simulink model "artigo_pista"  (R2018a)
settings: Solver=ode45  StartTime=0.0  StopTime=6  RelTol=1e-5  EnableMultiTasking=on
undefined symbols (not defined in the file): KIm, Km, KPm, mapa_pista_artigo, Pm, Ts
libraries: simulink x4
settings Model: Creator=dwbertol  LastModifiedBy=bruno
settings DataIOCC: LimitDataPoints=on  SaveFormat=Array  SignalLoggingSaveFormat=ModelDataLogs
settings OptimizationCC: ExpressionDepthLimit=2147483647  LifeSpan=inf
settings DebuggingCC: UnderspecifiedInitializationDetection=Classic  MergeDetectMultiDrivingBlocksExec=none  SolverPrmCheckMsg=warning  FcnCallInpInsideContextMsg=warning  StateNameClashWarn=warning  SFUnexpectedBacktrackingDiag=warning  SFNoUnconditionalDefaultTransitionDiag=warning  SFExecutionAtInitializationDiag=none
settings HardwareCC: ProdBitPerPointer=32  ProdBitPerSizeT=32  ProdBitPerPtrDiffT=32  ProdLargestAtomicFloat=None  ProdIntDivRoundTo=Undefined  ProdEndianess=Unspecified  ProdWordSize=32  ProdHWDeviceType=32-bit Generic
settings ModelReferenceCC: PropagateSignalLabelsOutOfModel=off
settings CodeAppCC: StateflowObjectComments=on
settings GRTTargetCC: TargetLangStandard=C89/C90 (ANSI)  GeneratePreprocessorConditionals=Disable all  CombineOutputUpdateFcns=off  GRTInterface=on
settings ConfigComp: CovMetricSettings=dw  CovHtmlReporting=on  CovSaveCumulativeToWorkspaceVar=on  CovSaveSingleToWorkspaceVar=on  CovExternalEMLEnable=off

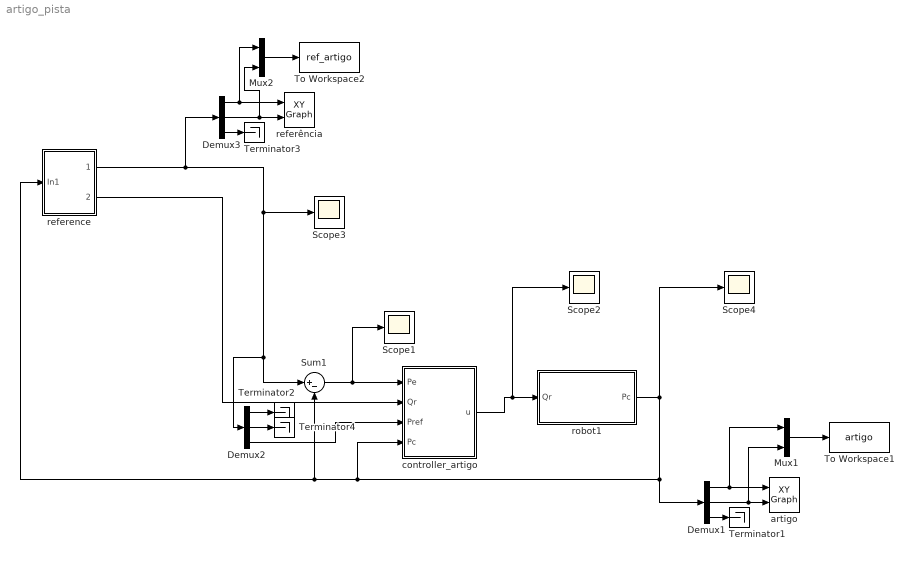
== system artigo_pista ==
  Demux1 : Demux  Outputs=3
  Demux2 : Demux  Outputs=3
  Demux3 : Demux  Outputs=3
  Mux1 : Mux  Inputs=2
  Mux2 : Mux  Inputs=2
  Scope{1..4} (4 alike) : Scope
  Sum1 : Sum  Inputs=|+-  AccumDataTypeStr=double
  Terminator{1..4} (4 alike) : Terminator
  To Workspace1 : ToWorkspace  VariableName=artigo  SampleTime=-1
  To Workspace2 : ToWorkspace  VariableName=ref_artigo  SampleTime=-1
  artigo : simulink/Sinks/XY Graph  xmin=-1.1  xmax=0.7  ymin=-0.1  ymax=1  st=Ts
  controller_artigo : Subsystem  mask{k1=400, k2=600}
  reference : Subsystem  mask{vr=1, wr=0, ini=[0 0.04 0], Ts=Ts}
  referência : simulink/Sinks/XY Graph  xmin=-1.1  xmax=0.7  ymin=-0.1  ymax=1  st=Ts
  robot1 : Subsystem  mask{ini=[0 0 0]'}
  wires:
  Demux1/1 -> Mux1/1, artigo/1
  Sum1/1 -> Scope1/1, controller_artigo/1(Pe)
  robot1/1(Pc) -> Scope4/1, Demux1/1, controller_artigo/4(Pc), reference/1(In1), Sum1/2
  Demux1/3 -> Terminator1/1
  controller_artigo/1(u) -> Scope2/1, robot1/1(Qr)
  Demux1/2 -> Mux1/2, artigo/2
  Demux3/1 -> Mux2/1, referência/1
  Demux3/3 -> Terminator3/1
  Demux3/2 -> Mux2/2, referência/2
  Mux1/1 -> To Workspace1/1
  reference/1("[xr yr tr]' ") -> Demux3/1, Scope3/1, Demux2/1, Sum1/1
  reference/2("[vr wr]'") -> controller_artigo/2(Qr)
  Mux2/1 -> To Workspace2/1
  Demux2/3 -> controller_artigo/3(Pref)
  Demux2/1 -> Terminator2/1
  Demux2/2 -> Terminator4/1

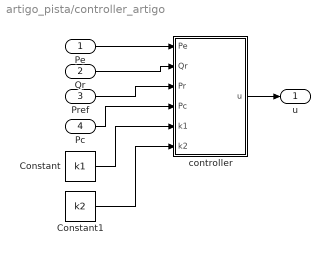
== system artigo_pista/controller_artigo ==
  Pe : Inport
  Qr : Inport  Port=2
  Pref : Inport  Port=3
  Pc : Inport  Port=4
  Constant : Constant  Value=k1
  Constant1 : Constant  Value=k2
  controller : MATLAB Function  TreatAsAtomicUnit=on
  u : Outport
  wires:
  Qr/1 -> controller/2(Qr)
  Pe/1 -> controller/1(Pe)
  controller/1(u) -> u/1
  Constant/1 -> controller/5(k1)
  Constant1/1 -> controller/6(k2)
  Pc/1 -> controller/4(Pc)
  Pref/1 -> controller/3(Pr)

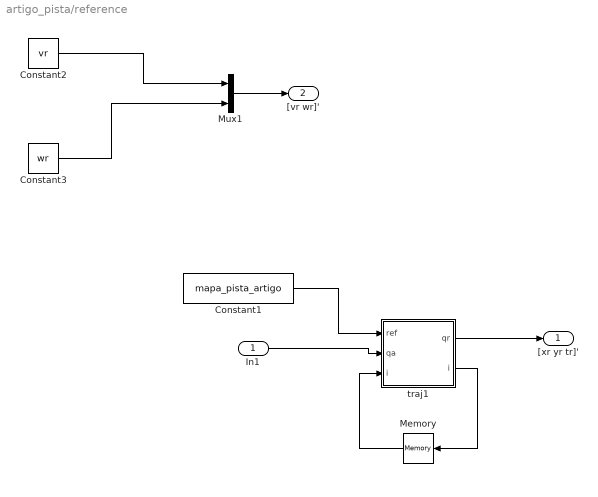
== system artigo_pista/reference ==
  In1 : Inport
  Constant1 : Constant  Value=mapa_pista_artigo
  Constant2 : Constant  Value=vr  VectorParams1D=off
  Constant3 : Constant  Value=wr  VectorParams1D=off
  Memory : Memory  InitialCondition=1
  Mux1 : Mux  Inputs=2
  traj1 : MATLAB Function  TreatAsAtomicUnit=on
  "[xr yr tr]' " : Outport
  "[vr wr]'" : Outport  Port=2
  wires:
  Constant3/1 -> Mux1/2
  Constant2/1 -> Mux1/1
  Mux1/1 -> "[vr wr]'"/1
  Constant1/1 -> traj1/1(ref)
  In1/1 -> traj1/2(qa)
  traj1/1(qr) -> "[xr yr tr]' "/1
  traj1/2(i) -> Memory/1
  Memory/1 -> traj1/3("i ")

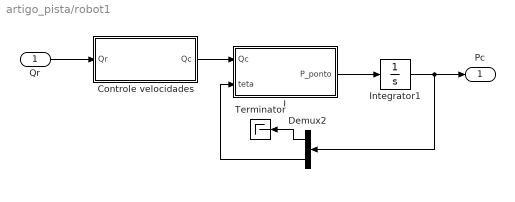
== system artigo_pista/robot1 ==
  Qr : Inport
  Controle velocidades : Subsystem
  Demux2 : Demux  Outputs=[2 1]
  Integrator1 : Integrator  InitialCondition=ini
  J : MATLAB Function  TreatAsAtomicUnit=on
  Terminator : Terminator
  Pc : Outport
  wires:
  J/1(P_ponto) -> Integrator1/1
  Integrator1/1 -> Demux2/1, Pc/1
  Demux2/1 -> Terminator/1
  Qr/1 -> Controle velocidades/1(Qr)
  Controle velocidades/1(Qc) -> J/1(Qc)
  Demux2/2 -> J/2(teta)

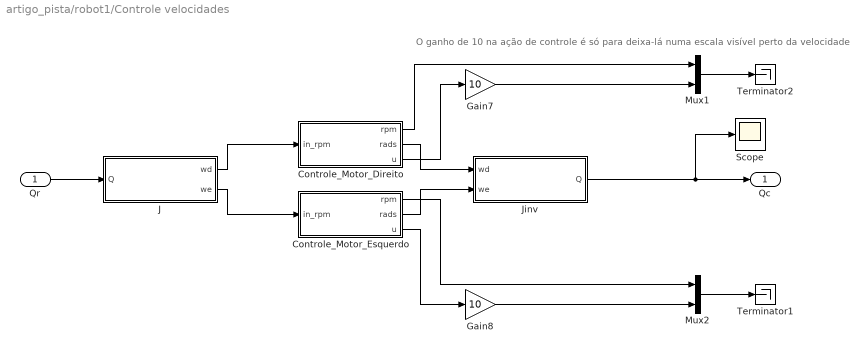
== system artigo_pista/robot1/Controle velocidades ==
  note: O ganho de 10 na ação de controle é só para deixa-lá numa escala visível perto da velocidade
  Qr : Inport
  Controle_Motor_Direito : Subsystem
  Controle_Motor_Esquerdo : Subsystem
  Gain7 : Gain  Gain=10
  Gain8 : Gain  Gain=10
  J : MATLAB Function  TreatAsAtomicUnit=on
  Jinv : MATLAB Function  TreatAsAtomicUnit=on
  Mux1 : Mux  Inputs=2
  Mux2 : Mux  Inputs=2
  Scope : Scope
  Terminator1 : Terminator
  Terminator2 : Terminator
  Qc : Outport
  wires:
  Gain7/1 -> Mux1/2
  Mux2/1 -> Terminator1/1
  Mux1/1 -> Terminator2/1
  Gain8/1 -> Mux2/2
  Controle_Motor_Direito/3(u) -> Gain7/1
  Controle_Motor_Direito/1(rpm) -> Mux1/1
  Controle_Motor_Esquerdo/3(u) -> Gain8/1
  Controle_Motor_Esquerdo/1(rpm) -> Mux2/1
  Qr/1 -> J/1(Q)
  J/1(wd) -> Controle_Motor_Direito/1(in_rpm)
  J/2(we) -> Controle_Motor_Esquerdo/1(in_rpm)
  Controle_Motor_Direito/2(rads) -> Jinv/1(wd)
  Controle_Motor_Esquerdo/2(rads) -> Jinv/2(we)
  Jinv/1(Q) -> Scope/1, Qc/1

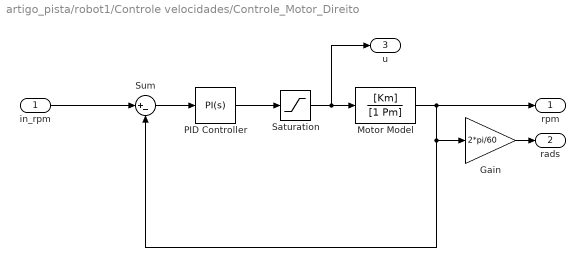
== system artigo_pista/robot1/Controle velocidades/Controle_Motor_Direito ==
  in_rpm : Inport
  Gain : Gain  Gain=2*pi/60
  Motor Model : TransferFcn  Numerator=[Km]  Denominator=[1 Pm]
  PID Controller : simulink/Continuous/PID Controller  Controller=PI  TimeDomain=Continuous-time  SampleTime=-1  IntegratorMethod=Forward Euler  FilterMethod=Forward Euler  Form=Parallel  UseFilter=on  ControllerParametersSource=internal  P=KPm  I=KIm  D=0  N=0  InitialConditionSource=internal  InitialConditionForIntegrator=0  InitialConditionForFilter=0  ExternalReset=none  LimitOutput=off  UpperSaturationLimit=inf  LowerSaturationLimit=-inf  LinearizeAsGain=on  AntiWindupMode=none  Kb=1  TrackingMode=off  Kt=1  PParamMin=[]  PParamMax=[]  IParamMin=[]  IParamMax=[]  DParamMin=[]  DParamMax=[]  NParamMin=[]  NParamMax=[]  KbParamMin=[]  KbParamMax=[]  KtParamMin=[]  KtParamMax=[]  POutMin=[]  POutMax=[]  IOutMin=[]  IOutMax=[]  DOutMin=[]  DOutMax=[]  NOutMin=[]  NOutMax=[]  KbOutMin=[]  KbOutMax=[]  KtOutMin=[]  KtOutMax=[]  IntegratorOutMin=[]  IntegratorOutMax=[]  FilterOutMin=[]  FilterOutMax=[]  SumOutMin=[]  SumOutMax=[]  SumI1OutMin=[]  SumI1OutMax=[]  SumI2OutMin=[]  SumI2OutMax=[]  SumI3OutMin=[]  SumI3OutMax=[]  SumDOutMin=[]  SumDOutMax=[]  SaturationOutMin=[]  SaturationOutMax=[]  IntegratorContinuousStateAttributes=''  IntegratorStateMustResolveToSignalObject=off  IntegratorRTWStateStorageClass=Auto  FilterContinuousStateAttributes=''  FilterStateMustResolveToSignalObject=off  FilterRTWStateStorageClass=Auto  DifferentiatorICPrevScaledInput=0  DifferentiatorOutMin=[]  DifferentiatorOutMax=[]  FilterDiffOutCoefMin=[]  FilterDiffOutCoefMax=[]  SumDenOutMin=[]  SumDenOutMax=[]  SumNumOutMin=[]  SumNumOutMax=[]  ReciprocalOutMin=[]  ReciprocalOutMax=[]  DivideOutMin=[]  DivideOutMax=[]  TunerSelectOption=Transfer Function Based (PID Tuner App)
  Saturation : Saturate  UpperLimit=100  LowerLimit=-100
  Sum : Sum  Inputs=|+-
  rpm : Outport
  rads : Outport  Port=2
  u : Outport  Port=3
  wires:
  PID Controller/1 -> Saturation/1
  Motor Model/1 -> rpm/1, Gain/1, Sum/2
  Saturation/1 -> u/1, Motor Model/1
  Sum/1 -> PID Controller/1
  in_rpm/1 -> Sum/1
  Gain/1 -> rads/1

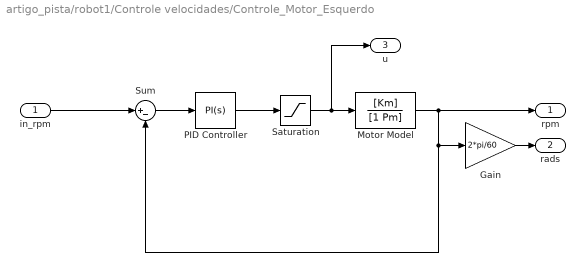
== system artigo_pista/robot1/Controle velocidades/Controle_Motor_Esquerdo ==
  in_rpm : Inport
  Gain : Gain  Gain=2*pi/60
  Motor Model : TransferFcn  Numerator=[Km]  Denominator=[1 Pm]
  PID Controller : simulink/Continuous/PID Controller  Controller=PI  TimeDomain=Continuous-time  SampleTime=-1  IntegratorMethod=Forward Euler  FilterMethod=Forward Euler  Form=Parallel  UseFilter=on  ControllerParametersSource=internal  P=KPm  I=KIm  D=0  N=0  InitialConditionSource=internal  InitialConditionForIntegrator=0  InitialConditionForFilter=0  ExternalReset=none  LimitOutput=off  UpperSaturationLimit=inf  LowerSaturationLimit=-inf  LinearizeAsGain=on  AntiWindupMode=none  Kb=1  TrackingMode=off  Kt=1  PParamMin=[]  PParamMax=[]  IParamMin=[]  IParamMax=[]  DParamMin=[]  DParamMax=[]  NParamMin=[]  NParamMax=[]  KbParamMin=[]  KbParamMax=[]  KtParamMin=[]  KtParamMax=[]  POutMin=[]  POutMax=[]  IOutMin=[]  IOutMax=[]  DOutMin=[]  DOutMax=[]  NOutMin=[]  NOutMax=[]  KbOutMin=[]  KbOutMax=[]  KtOutMin=[]  KtOutMax=[]  IntegratorOutMin=[]  IntegratorOutMax=[]  FilterOutMin=[]  FilterOutMax=[]  SumOutMin=[]  SumOutMax=[]  SumI1OutMin=[]  SumI1OutMax=[]  SumI2OutMin=[]  SumI2OutMax=[]  SumI3OutMin=[]  SumI3OutMax=[]  SumDOutMin=[]  SumDOutMax=[]  SaturationOutMin=[]  SaturationOutMax=[]  IntegratorContinuousStateAttributes=''  IntegratorStateMustResolveToSignalObject=off  IntegratorRTWStateStorageClass=Auto  FilterContinuousStateAttributes=''  FilterStateMustResolveToSignalObject=off  FilterRTWStateStorageClass=Auto  DifferentiatorICPrevScaledInput=0  DifferentiatorOutMin=[]  DifferentiatorOutMax=[]  FilterDiffOutCoefMin=[]  FilterDiffOutCoefMax=[]  SumDenOutMin=[]  SumDenOutMax=[]  SumNumOutMin=[]  SumNumOutMax=[]  ReciprocalOutMin=[]  ReciprocalOutMax=[]  DivideOutMin=[]  DivideOutMax=[]  TunerSelectOption=Transfer Function Based (PID Tuner App)
  Saturation : Saturate  UpperLimit=100  LowerLimit=-100
  Sum : Sum  Inputs=|+-
  rpm : Outport
  rads : Outport  Port=2
  u : Outport  Port=3
  wires:
  PID Controller/1 -> Saturation/1
  Saturation/1 -> u/1, Motor Model/1
  Sum/1 -> PID Controller/1
  in_rpm/1 -> Sum/1
  Motor Model/1 -> rpm/1, Gain/1, Sum/2
  Gain/1 -> rads/1

== matlab function artigo_pista/controller_artigo/controller ==
  data: Pe input; Qr input; Pr input; Pc input; k1 input; u output; k2 input
function u = fcn(Pe,Qr,Pr,Pc,k1,k2)

% Pe = -Pe;
% Pe = -[cos(Pc(3)) sin(Pc(3)) 0; -sin(Pc(3)) cos(Pc(3)) 0; 0 0 1]*Pe;
% Pe(2) = -Pe(2);
% 
% if Pe(3) ~= 0
%     w = k1*Pe(3) + k2*Pe(2)*Qr(1)*sin(Pe(3))/Pe(3);
% else
%     w = k2*Pe(2)*Qr(1);
% end
l = sin(Pr)*(Pe(1)) + cos(Pr)*(Pe(2));
if Pe(3) ~= 0
    w = k1*Pe(3) + k2*l*Qr(1)*sin(Pe(3))/Pe(3);
else
    w = k2*l*Qr(1);
end

u = [Qr(1); w];
 
end

== matlab function artigo_pista/robot1/Controle velocidades/J ==
  data: Q input; wd output; we output
function [wd, we] = fcn(Q)
% Dados do robô
r = 16e-3;      % Raio da roda
a = 69e-3;      % Distância do centro do robô até o centro das rodas

w_mot_rpm = (60/(2*pi))*[1/r a/r; 1/r -a/r]*Q;   % o 60/(2pi) é pra converter p/ rpm
wd = w_mot_rpm(1);
we = w_mot_rpm(2);

== matlab function artigo_pista/robot1/Controle velocidades/Jinv ==
  data: wd input; Q output; we input
function Q = fcn(wd, we)
% Dados do robô
r = 16e-3;      % Raio da roda
a = 69e-3;      % Distância do centro do robô até o centro das rodas

Q = (r/2)*[1 1; 1/a -1/a]*[wd; we];

== matlab function artigo_pista/robot1/J ==
  data: Qc input; P_ponto output; teta input
function P_ponto = fcn(Qc, teta)

P_ponto = [Qc(1)*cos(teta); Qc(1)*sin(teta); Qc(2)]; %[Vx, Vy, Vteta];

== matlab function artigo_pista/reference/traj1 ==
  data: ref input; qa input; qr output; i input; i output
function [qr, i] = fcn(ref, qa, i)

    A = [ones(100,1)*qa(1), ones(100,1)*qa(2)];
    
    B = ref(i:i+99,1:2);
    %compute Euclidean distances:
    dist2 = sum((B - A) .^ 2, 2);
    %find the smallest distance and use that as an index into B:
    [v, idx] = min(dist2);
    qr = ref(i+idx-1,:);    

    i = i+idx-1;
    %qr = [1 2 3];
 
end
